simulink model "pendcart_remodel"  (Simulink 8.9)
settings: Solver=ode45  StartTime=0.0  StopTime=tsim  RelTol=1e-3  EnableMultiTasking=on
values from neighbouring files (symbols this model uses):
  b = 0.01    [pendcartsim.m]
  c = 0.05    [pendcartsim.m]
  g = 9.82    [pendcartsim.m]
  K1 = -119.0071    [pendcartsim.m]
  K2 = 0.0402    [pendcartsim.m]
  l = 0.5    [pendcartsim.m]
  M = 1    [pendcartsim.m]
  m = 0.5    [pendcartsim.m]
  p = 5.4277    [pendcartsim.m]
  p1 = 25.4277    [pendcartsim.m]
  theta0 = 5*pi/180    (= 0.0872664625997)    [pendcartsim.m]
  Wheel_Radius = 0.035    [pendcartsim.m]
undefined symbols (not defined in the file or in its folder): sigbuilder_block
settings Model: Creator=Chris  LastModifiedBy=Administrator
settings OptimizationCC: ExpressionDepthLimit=2147483647  InitFltsAndDblsToZero=on
settings DebuggingCC: AlgebraicLoopMsg=none  SaveWithParameterizedLinksMsg=none
settings GRTTargetCC: TargetFcnLib=ansi_tfl_tmw.mat

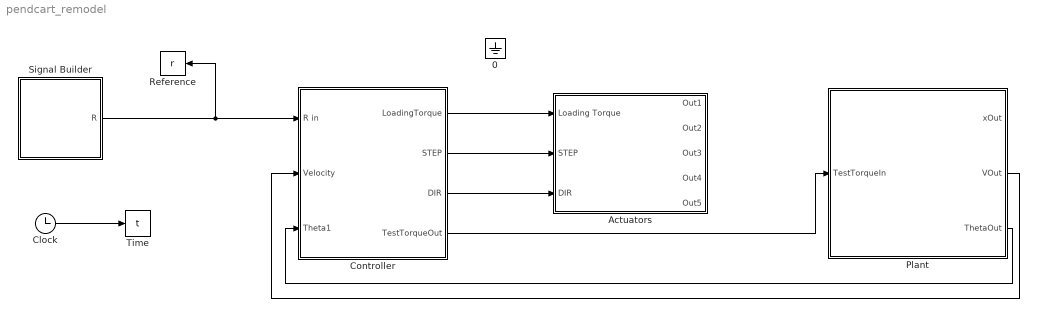
== system pendcart_remodel ==
  0 : Ground
  Actuators : Subsystem
  Clock : Clock
  Controller : Subsystem
  Plant : Subsystem
  Reference : ToWorkspace  VariableName=r  SampleTime=-1
  Signal Builder : Subsystem  Tag=STV Subsys  LoadFcn=sigbuilder_block('load');  StartFcn=sigbuilder_block('start');  StopFcn=sigbuilder_block('stop');  ClipboardFcn=sigbuilder_block('clipboard');  mask(Sigbuilder block){tuvar=[0:10]}
      mask help: Sigbuilder GUI
      mask init:
      | if ~strcmp(get_param(bdroot(gcbh),'SimulationStatus'),'stopped') tuvar = sigbuilder_block('maskInit'); end
      settings: CopyFcn=sigbuilder_block('copy');  DeleteFcn=sigbuilder_block('delete');  ModelCloseFcn=sigbuilder_block('modelClose');  PreSaveFcn=sigbuilder_block('preSave');  PauseFcn=sigbuilder_block('pause')  ContinueFcn=sigbuilder_block('continue')  NameChangeFcn=sigbuilder_block('namechange');  OpenFcn=sigbuilder_block('open',[5.5 23 949 425 ]);  CloseFcn=sigbuilder_block('close');
      mask Display: plot(0, 0, 100, 100,[2, 2, 32, 32, 2], [68, 8, 8, 68, 68],[32, 2], [38, 38], [32, 19, 2],[53, 60, 44], [32, 17, 17, 2],[16, 16, 31, 31]);txt = getActiveGroup(gcbh);text(2, 100, txt,'verticalAlignment', 'top');
  Time : ToWorkspace  VariableName=t  SampleTime=-1
  wires:
  Clock/1 -> Time/1
  Plant/2(VOut) -> Controller/2(Velocity)
  Signal Builder/1(R) -> Controller/1(R in), Reference/1
  Controller/4(TestTorqueOut) -> Plant/1(TestTorqueIn)
  Plant/3(ThetaOut) -> Controller/3(Theta1)
  Controller/3(DIR) -> Actuators/3(DIR)
  Controller/1(LoadingTorque) -> Actuators/1(Loading Torque)
  Controller/2(STEP) -> Actuators/2(STEP)

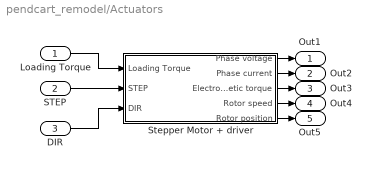
== system pendcart_remodel/Actuators ==
  Loading Torque : Inport
  STEP : Inport  Port=2
  DIR : Inport  Port=3
  Stepper Motor + driver : Subsystem
  Out1 : Outport
  Out2 : Outport  Port=2
  Out3 : Outport  Port=3
  Out4 : Outport  Port=4
  Out5 : Outport  Port=5
  wires:
  Stepper Motor + driver/3(Electromagnetic torque) -> Out3/1
  Stepper Motor + driver/2(Phase current) -> Out2/1
  Stepper Motor + driver/4(Rotor speed) -> Out4/1
  Stepper Motor + driver/5(Rotor position) -> Out5/1
  Stepper Motor + driver/1(Phase voltage) -> Out1/1
  STEP/1 -> Stepper Motor + driver/2(STEP)
  DIR/1 -> Stepper Motor + driver/3(DIR)
  Loading Torque/1 -> Stepper Motor + driver/1(Loading Torque)

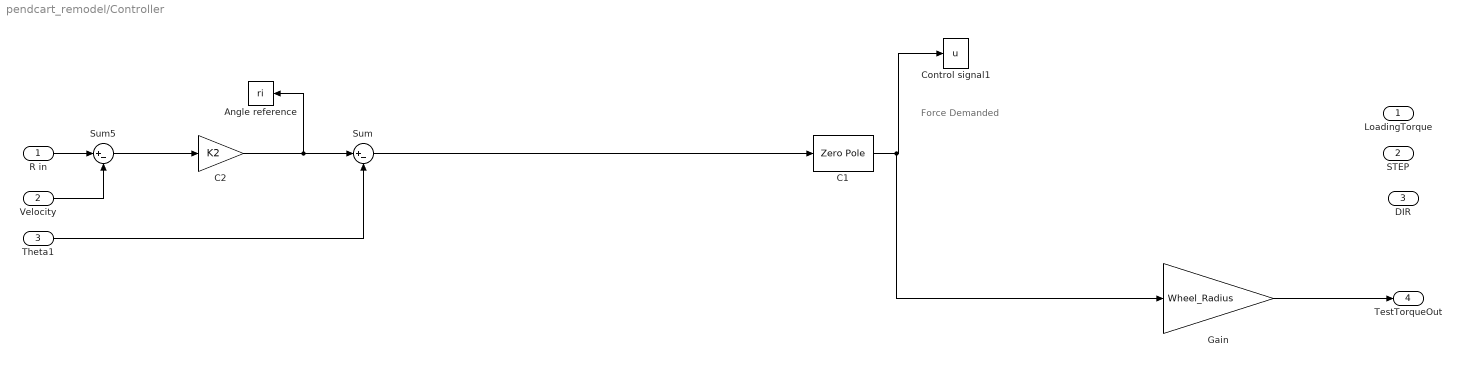
== system pendcart_remodel/Controller ==
  note: Force Demanded
  R in : Inport
  Velocity : Inport  Port=2
  Theta1 : Inport  Port=3
  Angle reference : ToWorkspace  VariableName=ri  SampleTime=-1
  C1 : ZeroPole  Zeros=[-p]  Poles=[-p1]  Gain=[K1]
  C2 : Gain  Gain=K2
  Control signal1 : ToWorkspace  VariableName=u  SampleTime=-1
  Gain : Gain  Gain=Wheel_Radius
  Sum : Sum  Inputs=|+-
  Sum5 : Sum  Inputs=|+-
  LoadingTorque : Outport
  STEP : Outport  Port=2
  DIR : Outport  Port=3
  TestTorqueOut : Outport  Port=4
  wires:
  C1/1 -> Gain/1, Control signal1/1
  Sum/1 -> C1/1
  Gain/1 -> TestTorqueOut/1
  Sum5/1 -> C2/1
  Velocity/1 -> Sum5/2
  C2/1 -> Angle reference/1, Sum/1
  R in/1 -> Sum5/1
  Theta1/1 -> Sum/2

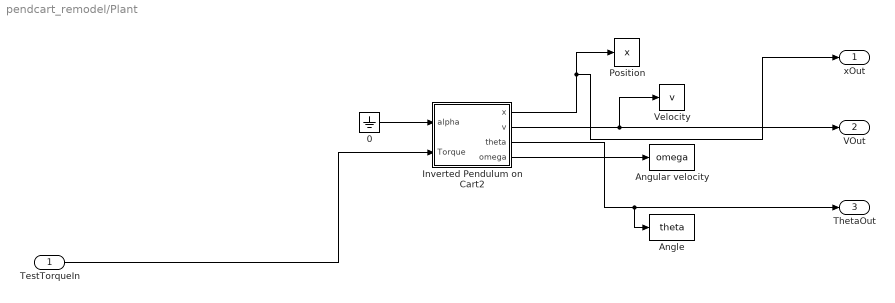
== system pendcart_remodel/Plant ==
  TestTorqueIn : Inport
  0 : Ground
  Angle : ToWorkspace  VariableName=theta  SampleTime=-1
  Angular velocity : ToWorkspace  VariableName=omega  SampleTime=-1
  Inverted Pendulum on Cart2 : Subsystem
  Position : ToWorkspace  VariableName=x  SampleTime=-1
  Velocity : ToWorkspace  VariableName=v  SampleTime=-1
  xOut : Outport
  VOut : Outport  Port=2
  ThetaOut : Outport  Port=3
  wires:
  Inverted Pendulum on Cart2/4(omega) -> Angular velocity/1
  Inverted Pendulum on Cart2/1(x) -> xOut/1, Position/1
  Inverted Pendulum on Cart2/3(theta) -> ThetaOut/1, Angle/1
  Inverted Pendulum on Cart2/2(v) -> VOut/1, Velocity/1
  0/1 -> Inverted Pendulum on Cart2/1(alpha)
  TestTorqueIn/1 -> Inverted Pendulum on Cart2/2(Torque)

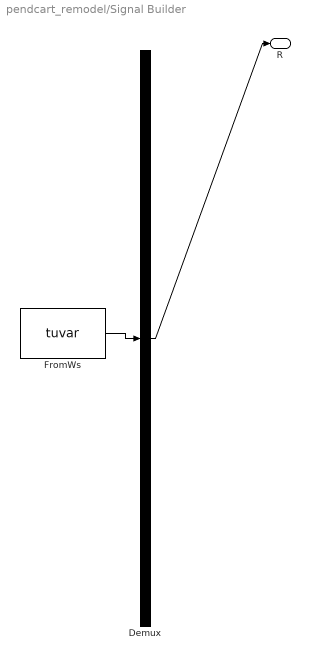
== system pendcart_remodel/Signal Builder ==
  Demux : Demux  Tag=STV Demux  Outputs=1
  FromWs : FromWorkspace  Tag=STV FromWs  VariableName=tuvar  SampleTime=0  SigBuilderData=DataTag0  VnvData=DataTag1
      SigBuilderData=|
      | common.afterFinalStr = 'Extrapolate'
      | common.sampleTime = 0
      | dataSet.timeRange = [0 20]
      | dataSet.name = 'Group 1'
      | sbobj.Groups.Name = 'Group 1'
      | sbobj.Groups.Signals.Name = 'R'
      | sbobj.Groups.Signals.XData = [0 8 8 12 12 20]
      | sbobj.Groups.Signals.YData = [0 0.48 1 1 0 0]
      | sbobj.Groups.TimeRange = [0 20]
  R : Outport  Tag=STV Outport
  wires:
  FromWs/1 -> Demux/1
  Demux/1 -> R/1

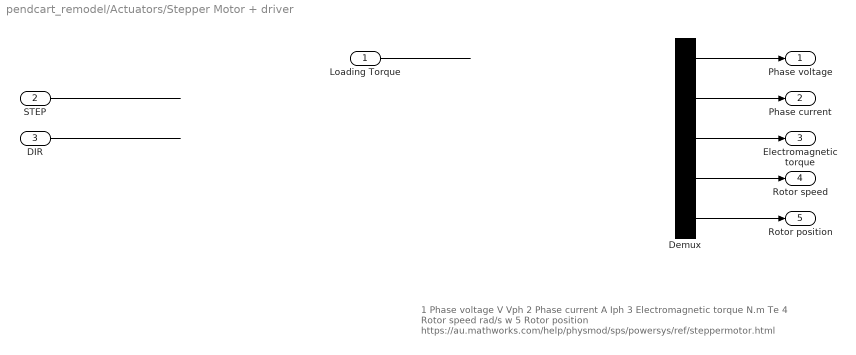
== system pendcart_remodel/Actuators/Stepper Motor + driver ==
  note: 1
      | Phase voltage
      | V
      | Vph
      |
      | 2
      | Phase current
      | A
      | Iph
      |
      | 3
      | Electromagnetic torque
      | N.m
      | Te
      |
      | 4
      | Rotor speed
      | rad/s
      | w
      |
      | 5
      | Rotor position
      |
      | https://au.mathworks.com/help/physmod/sps/powersys/ref/steppermotor.html
  Loading Torque : Inport
  STEP : Inport  Port=2
  DIR : Inport  Port=3
  Demux : Demux  Outputs=5
  Phase voltage : Outport
  Phase current : Outport  Port=2
  Electromagnetic torque : Outport  Port=3
  Rotor speed : Outport  Port=4
  Rotor position : Outport  Port=5
  wires:
  Demux/2 -> Phase current/1
  Loading Torque/1 -> ?
  Demux/3 -> Electromagnetic torque/1
  Demux/1 -> Phase voltage/1
  Demux/4 -> Rotor speed/1
  ? -> Demux/1
  Demux/5 -> Rotor position/1
  DIR/1 -> ?
  STEP/1 -> ?

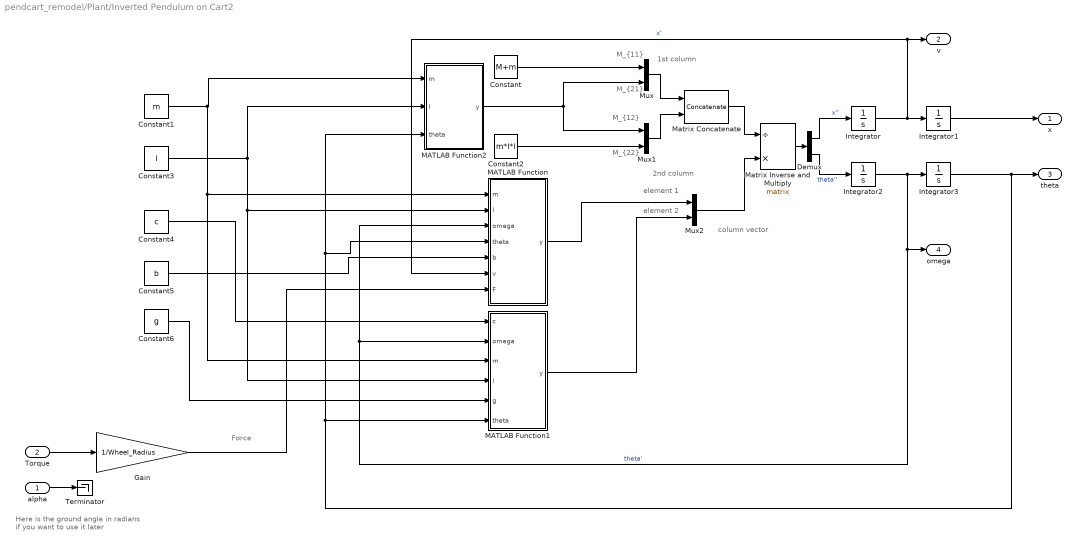
== system pendcart_remodel/Plant/Inverted Pendulum on Cart2 ==
  note: Force
  note: 2nd column
  note: M_{21}
  note: 1st column
  note: M_{12}
  note: element 2
  note: Here is the ground angle in
      | radians if you want to use it later
  note: column vector
  note: M_{11}
  note: M_{22}
  note: element 1
  alpha : Inport
  Torque : Inport  Port=2
  Constant : Constant  Value=M+m
  Constant1 : Constant  Value=m
  Constant2 : Constant  Value=m*l*l
  Constant3 : Constant  Value=l
  Constant4 : Constant  Value=c
  Constant5 : Constant  Value=b
  Constant6 : Constant  Value=g
  Demux : Demux  Outputs=2
  Gain : Gain  Gain=1/Wheel_Radius
  Integrator : Integrator
  Integrator1 : Integrator
  Integrator2 : Integrator
  Integrator3 : Integrator  InitialCondition=theta0
  MATLAB Function : MATLAB Function  TreatAsAtomicUnit=on
  MATLAB Function1 : MATLAB Function  TreatAsAtomicUnit=on
  MATLAB Function2 : MATLAB Function  TreatAsAtomicUnit=on
  Matrix Concatenate : Concatenate  Mode=Multidimensional array  ConcatenateDimension=2
  Matrix Inverse and Multiply : Product  Inputs=/*  Multiplication=Matrix(*)
  Mux : Mux  Inputs=2
  Mux1 : Mux  Inputs=2
  Mux2 : Mux  Inputs=2
  Terminator : Terminator
  x : Outport
  v : Outport  Port=2
  theta : Outport  Port=3
  omega : Outport  Port=4
  wires:
  MATLAB Function1/1(y) -> Mux2/2
  Constant1/1 -> MATLAB Function1/3(m), MATLAB Function/1(m), MATLAB Function2/1(m)
  Constant5/1 -> MATLAB Function/5(b)
  Matrix Inverse and Multiply/1 -> Demux/1
  Constant2/1 -> Mux1/2
  Mux2/1 -> Matrix Inverse and Multiply/2
  MATLAB Function/1(y) -> Mux2/1
  Constant4/1 -> MATLAB Function1/1(c)
  Mux1/1 -> Matrix Concatenate/2
  Constant/1 -> Mux/1
  MATLAB Function2/1(y) -> Mux1/1, Mux/2
  Integrator/1 -> Integrator1/1, v/1, MATLAB Function/6(v)  "x'"
  Matrix Concatenate/1 -> Matrix Inverse and Multiply/1
  Integrator1/1 -> x/1
  Demux/2 -> Integrator2/1  "theta''"
  Integrator3/1 -> MATLAB Function/4(theta), MATLAB Function2/3(theta), MATLAB Function1/6(theta), theta/1
  Constant3/1 -> MATLAB Function1/4(l), MATLAB Function/2(l), MATLAB Function2/2(l)
  Mux/1 -> Matrix Concatenate/1
  Integrator2/1 -> Integrator3/1, MATLAB Function/3(omega), MATLAB Function1/2(omega), omega/1  "theta'"
  Constant6/1 -> MATLAB Function1/5(g)
  alpha/1 -> Terminator/1
  Demux/1 -> Integrator/1  "x''"
  Torque/1 -> Gain/1
  Gain/1 -> MATLAB Function/7(F)

== matlab function Plant/Inverted Pendulum on Cart2/MATLAB Function1 ==
  data: y output double; c input double; omega input double; m input double; l input double; g input double; theta input double
function y  = fcn(c,omega,m,l,g,theta)

y =c*omega+m*l*g*sin(theta);

== matlab function Plant/Inverted Pendulum on Cart2/MATLAB Function ==
  data: y output double; m input double; l input double; omega input double; theta input double; b input double; v input double; F input double
function y = fcn(m,l,omega,theta,b,v,F)

y =m*l*omega*omega*sin(theta)+b*v+F;

== matlab function Plant/Inverted Pendulum on Cart2/MATLAB Function2 ==
  data: y output double; m input double; l input double; theta input double
function y = fcn(m,l,theta)

y =m*l*cos(theta);
